simulink model "problem1"  (R2020b)
settings: Solver=VariableStepAuto  StartTime=0.0  StopTime=10.0  RelTol=1e-3
settings Model: Creator=admin  LastModifiedBy=admin

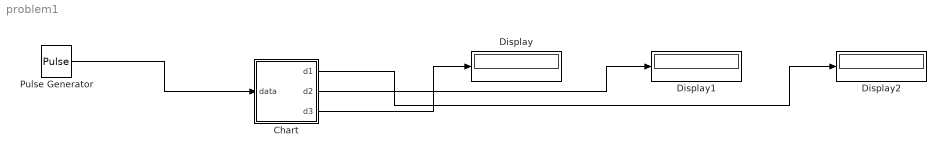
== system problem1 ==
  Chart : Stateflow chart  TreatAsAtomicUnit=on
  Display : Display
  Display1 : Display
  Display2 : Display
  Pulse Generator : DiscretePulseGenerator  PulseType=Time based  Period=10  PulseWidth=5
  wires:
  Pulse Generator/1 -> Chart/1(data)
  Chart/1(d1) -> Display2/1
  Chart/2(d2) -> Display1/1
  Chart/3(d3) -> Display/1

== stateflow chart problem1/Chart ==
  state one
    en:
    d1=1
  state zero
    en:
    d1=0;
  state two
    en:
    d1=2;
  state four
    en:
    d1=4;
  state three
    en:
    d1=3;
  state one1
    en:
    d2=1
  state zero1
    en:
    d2=0;
  state two1
    en:
    d2=2
  state four1
    en:
    d2=4;
  state three1
    en:
    d2=3;
  state one2
    en:
    d3=1
  state two2
    en:
    d3=2;
  state zero2
    en:
    d3=0;
  state four2
    en:
    d4=4;
  state three2
    en:
    d3=3;
  one -> two : inc3
  (default) -> zero [order 3]
  zero -> one : inc1
  four -> zero
  two -> three : inc3
  three -> four : inc1
  one1 -> two1 : inc2
  zero1 -> one1 : inc2
  (default) -> zero1 [order 1]
  four1 -> zero1 : inc2
  two1 -> three1 : inc2
  three1 -> four1 : inc2
  one2 -> two2 : inc3
  zero2 -> one2 : inc3
  (default) -> zero2 [order 2]
  two2 -> three2 : inc3
  four2 -> zero2 : inc3
  three2 -> four2 : inc3
  data: d1 output; d2 output; d3 output; data input
  events: inc1 local FUNCTION_CALL_EVENT; inc3 local FUNCTION_CALL_EVENT; inc2 local FUNCTION_CALL_EVENT
